simulink model "lesson140313"  (R2013a)
settings: Solver=ode45  StartTime=0.0  StopTime=30.0  RelTol=1e-3
settings Model: Creator=mulleda2  LastModifiedBy=mulleda2

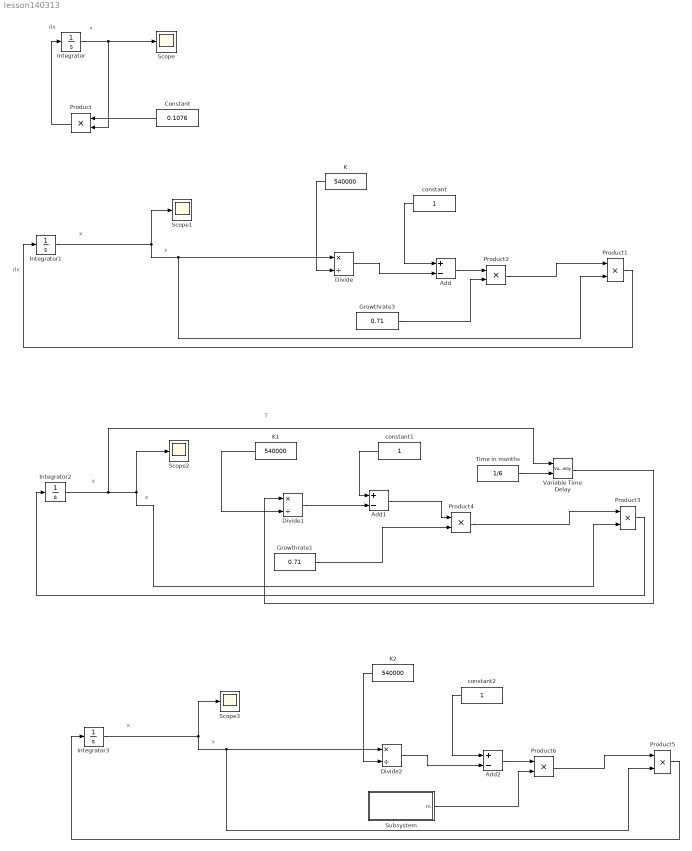
== system lesson140313 ==
  note: T
  note: x
  note: dx
  note: x
  note: x
  note: dx
  note: x
  note: x
  note: x
  note: x
  Add : Sum  Inputs=+-
  Add1 : Sum  Inputs=+-
  Add2 : Sum  Inputs=+-
  Constant : Constant  Value=0.1076
  Divide : Product  Inputs=*/
  Divide1 : Product  Inputs=*/
  Divide2 : Product  Inputs=*/
  Growthrate1 : Constant  Value=0.71
  Growthrate3 : Constant  Value=0.71
  Integrator : Integrator  InitialCondition=16.4775
  Integrator1 : Integrator  InitialCondition=540000/4
  Integrator2 : Integrator  InitialCondition=540000/4
  Integrator3 : Integrator  InitialCondition=540000/4
  K : Constant  Value=540000
  K1 : Constant  Value=540000
  K2 : Constant  Value=540000
  Product{,1..6} (7 alike) : Product
  Scope{,1..3} (4 alike) : Scope
      Scope2 settings: SaveName=ScopeData2
      Scope3 settings: SaveName=ScopeData3
  Subsystem : Subsystem
  Time in months : Constant  Value=1/6
  Variable Time Delay : VariableTransportDelay  MaximumDelay=10
  constant : Constant
  constant1 : Constant
  constant2 : Constant
  wires:
  Product/1 -> Integrator/1
  Integrator/1 -> Product/2, Scope/1
  Constant/1 -> Product/1
  Integrator1/1 -> Product1/2, Divide/1, Scope1/1
  K/1 -> Divide/2
  constant/1 -> Add/1
  Divide/1 -> Add/2
  Add/1 -> Product2/1
  Growthrate3/1 -> Product2/2
  Product2/1 -> Product1/1
  Product1/1 -> Integrator1/1
  Integrator2/1 -> Variable Time Delay/1, Product3/2, Scope2/1
  K1/1 -> Divide1/2
  constant1/1 -> Add1/1
  Divide1/1 -> Add1/2
  Add1/1 -> Product4/1
  Growthrate1/1 -> Product4/2
  Product4/1 -> Product3/1
  Product3/1 -> Integrator2/1
  Time in months/1 -> Variable Time Delay/2
  Variable Time Delay/1 -> Divide1/1
  Integrator3/1 -> Product5/2, Divide2/1, Scope3/1
  K2/1 -> Divide2/2
  constant2/1 -> Add2/1
  Divide2/1 -> Add2/2
  Add2/1 -> Product6/1
  Subsystem/1(ro) -> Product6/2
  Product6/1 -> Product5/1
  Product5/1 -> Integrator3/1

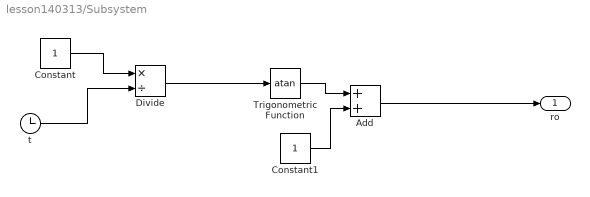
== system lesson140313/Subsystem ==
  Add : Sum
  Constant : Constant
  Constant1 : Constant
  Divide : Product  Inputs=*/
  Trigonometric Function : Trigonometry  Operator=atan
  "t " : Clock
  ro : Outport
  wires:
  Constant/1 -> Divide/1
  "t "/1 -> Divide/2
  Divide/1 -> Trigonometric Function/1
  Trigonometric Function/1 -> Add/1
  Constant1/1 -> Add/2
  Add/1 -> ro/1
